simulink model "DASHBOARDout"  (R2024a)
settings: Solver=VariableStepAuto  StartTime=0.0  StopTime=10.0  RelTol=1e-3
undefined symbols (not defined in the file or in its folder): canChannel
libraries: canlib x2, canmsglib x2
(part 1 of 2)
settings Model: DataDictionary=BMS_System_dict1.sldd  Creator=hirah  LastModifiedBy=hirah

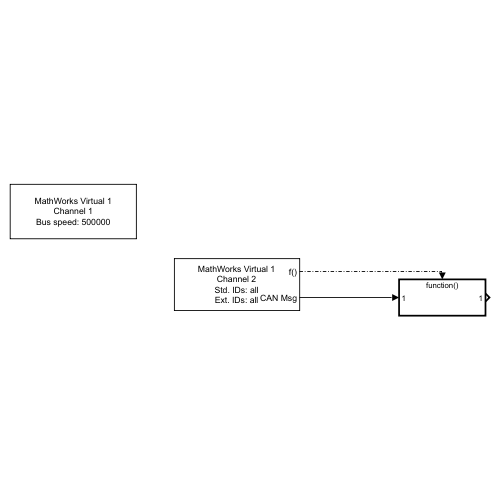
[thumbnail: Simulink's stored preview of the top-level diagram]
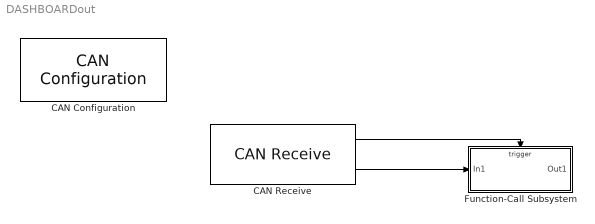
== system DASHBOARDout ==
  CAN Configuration : canlib/CAN Configuration  BlockHandle=570.0001  Device=MathWorks Virtual 1 (Channel 1)  DeviceMenu=MathWorks Virtual 1 (Channel 1)  ObjConstructor=canChannel('MathWorks', 'Virtual 1', 1)  BusSpeed=500000  EnableBitParameters=off  AckMode=Normal
  CAN Receive : canlib/CAN Receive  BlockHandle=729.0002  Device=MathWorks Virtual 1 (Channel 2)  DeviceMenu=MathWorks Virtual 1 (Channel 2)  ObjConstructor=canChannel('MathWorks', 'Virtual 1', 2)  EnableStandardIDsFilter=off  StdIDsCombo=Allow all  StandardIDs=261  EnableExtendedIDsFilter=off  ExtIDsCombo=Allow all  ExtendedIDs=0  SampleTime=0.01  MsgsPerTimestep=all  InternalFilterUpdateStatus=on  BusOutput=off
  Function-Call Subsystem : Subsystem  TreatAsAtomicUnit=on
  wires:
  CAN Receive/2 -> Function-Call Subsystem/1(In1)
  CAN Receive/1 -> Function-Call Subsystem/Trigger
